simulink model "Reaching"  (R2022b)
settings: Solver=FixedStepDiscrete  StartTime=0.0  StopTime=inf  FixedStep=0.001  RelTol=1e-3
libraries: PhanTorque_3Dof_Library_64Bits x1, vrlib x1
settings Model: Creator=carlos.aldana  LastModifiedBy=bioen
settings SolverCC: AlgebraicLoopSolver=TrustRegion
settings DataIOCC: LimitDataPoints=on  SaveFormat=Array  ReturnWorkspaceOutputs=off
settings OptimizationCC: BlockReduction=off  BooleanDataType=off  LifeSpan=inf
settings DebuggingCC: SaveWithParameterizedLinksMsg=none  UnderspecifiedInitializationDetection=Classic  MergeDetectMultiDrivingBlocksExec=none  SignalResolutionControl=TryResolveAllWithWarning  UnconnectedInputMsg=warning  UnconnectedOutputMsg=warning  UnconnectedLineMsg=warning  AllowSymbolicDim=off  SFUnexpectedBacktrackingDiag=warning  SFNoUnconditionalDefaultTransitionDiag=warning  SFExecutionAtInitializationDiag=none  SFMachineParentedDataDiag=warning  ArithmeticOperatorsInVariantConditions=warning
settings HardwareCC: ProdBitPerPointer=32  ProdBitPerSizeT=32  ProdBitPerPtrDiffT=32  ProdLargestAtomicFloat=None  ProdIntDivRoundTo=Undefined  ProdEndianess=Unspecified  ProdWordSize=32  ProdHWDeviceType=32-bit Generic  TargetUnknown=on
settings ModelReferenceCC: EnableRefExpFcnMdlSchedulingChecks=on  PropagateSignalLabelsOutOfModel=off
settings SFSimCC: SimUseLocalCustomCode=off  CustomCodeUndefinedFunction=UseInterfaceOnly
settings RTWCC: RTWUseLocalCustomCode=off  DLArmComputeVersion=19.05
settings CodeAppCC: StateflowObjectComments=on
settings GRTTargetCC: TargetLangStandard=C89/C90 (ANSI)
settings ConfigComp: CovMetricSettings=dw  CovSaveCumulativeToWorkspaceVar=on  CovSaveSingleToWorkspaceVar=on  CovExternalEMLEnable=off  CovSFcnEnable=off

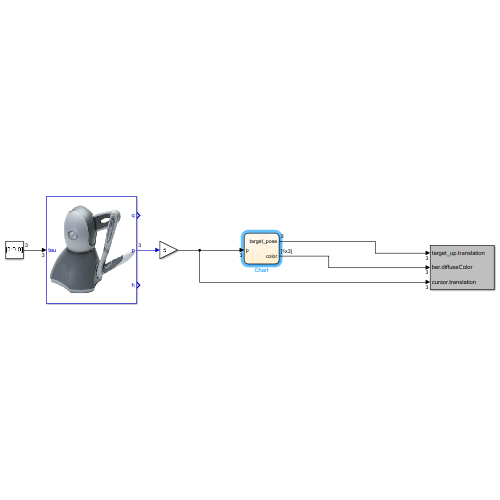
[thumbnail: Simulink's stored preview of the top-level diagram]
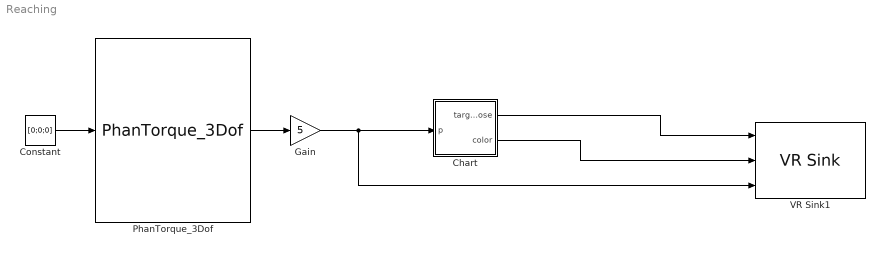
== system Reaching ==
  Chart : Stateflow chart  TreatAsAtomicUnit=on
  Constant : Constant  Value=[0;0;0]
  Gain : Gain  Gain=5
  PhanTorque_3Dof : PhanTorque_3Dof_Library_64Bits/PhanTorque_3Dof  Haptic_Name='Default Device'
  VR Sink1 : vrlib/VR Sink  InstantiateOnLoad=on  SampleTime=0.1  ViewEnable=on  RemoteChange=off  RemoteView=off  FieldsWritten=target_up.translation.3.1.1.double#ber.diffuseColor.3.1.1.double#cursor.translation.3.1.1.double  WorldFileName=8_palline_color.wrl  AutoView=off  VideoDimensions=[]  AllowVariableSize=off  FigureProperties="{'Position', 'Name', 'Viewpoint', 'CameraBound', 'CameraDirection', 'CameraPosition', 'CameraUpVector', 'ZoomFactor', 'Antialiasing', 'Headlight', 'Lighting', 'NavPanel', 'Sound', 'StatusBar', 'Stereo3D', 'Stereo3DCameraOffset', 'Stereo3DHIT', 'ToolBar', 'Textures', 'Transparency', 'Triad', 'Wireframe', 'NavZones', 'NavMode', 'NavSpeed', 'CaptureFileFormat', 'CaptureFileName', 'Record2DCompressMethod', 'Record2DCompressQuality', 'Record2D', 'Record2DFileName', 'Record2DFPS'; [8.2100000000000000e+02   3.0100000000000000e+02   5.7600000000000000e+02   3.5000000000000000e+02], '', '_untitled_1', 'on', [0.0000000000000000e+00   0.0000000000000000e+00  -1.0000000000000000e+00], [0.0000000000000000e+00   0.0000000000000000e+00   0.0000000000000000e+00], [0.0000000000000000e+00   1.0000000000000000e+00   0.0000000000000000e+00], [1.0000000000000000e+00], 'on', 'on', 'on', 'halfbar', 'on', 'on', 'off', [1.0000000149011612e-01], [0.0000000000000000e+00], 'on', 'on', 'on', 'none', 'off', 'off', 'fly', 'normal', 'tif', '%f_anim_%n.tif', 'auto', [7.5000000000000000e+01], 'off', '%f_anim_%n.avi', 'auto'}"
  wires:
  Constant/1 -> PhanTorque_3Dof/1
  Chart/2(color) -> VR Sink1/2
  Chart/1(target_pose) -> VR Sink1/1
  PhanTorque_3Dof/2 -> Gain/1
  Gain/1 -> VR Sink1/3, Chart/1(p)

== stateflow chart Reaching/Chart ==
  state initial
    entry:
    radius=0.1;
    counter=0;
    time=0;
    angle_matrix=[0 pi/4 pi/2 3/4*pi pi 5/4*pi 3/2*pi 7/4*pi];
  state rand_angle
    angle = angle_matrix(randi(8));
  state new_target
    entry:
    color=[1 0 0];
    target_pose=radius*[cos(angle); sin(angle); 0];
    err=norm(p(1:2)-target_pose(1:2));
    during:
    err=norm(p(1:2)-target_pose(1:2));
  state feedback
    entry:
    color=[0 0 1];
    during:
    err=norm(p(1:2)-target_pose(1:2));
  state back
    entry:
    target_pose=[0 0 0]';
    color=[1 0 0];
    during:
    err=norm(p(1:2)-target_pose(1:2));
  state feedback2
    entry:
    color=[0 0 1];
    during:
    err=norm(p(1:2)-target_pose(1:2));
  state finish
    end
  (default) -> initial
  initial -> rand_angle
  feedback2 -> rand_angle [order 1] : [err<0.01 & after (2, sec)]
  rand_angle -> new_target
  feedback -> new_target [order 2] : [err>=0.01]
  new_target -> feedback : [err<0.01]
  feedback -> back [order 1] : [err<0.01 & after(1, sec)]{counter = counter+1;}
  feedback2 -> back [order 2] : [err>=0.01]
  back -> feedback2 : [err<0.01]
  feedback2 -> finish [order 3] : [counter>=10]
  data: p input; target_pose output; color output; time local; angle_matrix local; angle local; counter local; err local; radius local
